simulink model "lqr_control_kalman_observer"  (R2020b)
settings: Solver=VariableStepAuto  StartTime=0.0  StopTime=30  RelTol=1e-3
undefined symbols (not defined in the file): A, B, C, C_discrete, D, D_discrete, DiscIntNeverNeededParam, Discrete, G, Gamma, h, h_plant, N, n, Phi, Q, Q0, Q1, Q2, R, R_discrete, reference, sat_max, sat_min, Time, wind_final_value, wind_initial_value, wind_steptime, x0
libraries: ctrlSharedLib x1
settings Model: Creator=lucas  LastModifiedBy=lucas

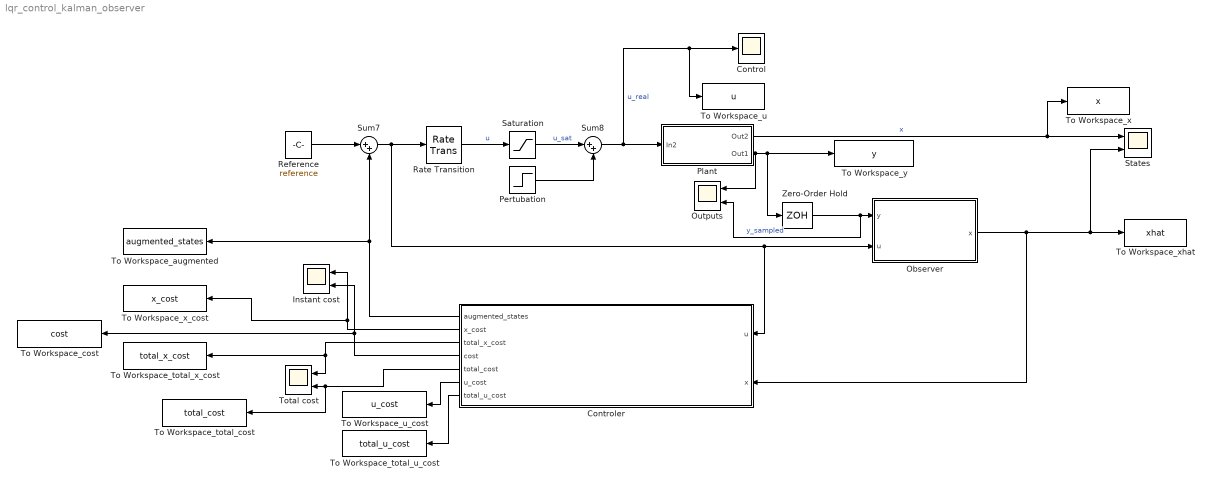
== system lqr_control_kalman_observer ==
  Control : Scope
  Controler : Subsystem
  Instant cost : Scope  NumInputPorts=2
  Observer : Subsystem
  Outputs : Scope  NumInputPorts=2
  Pertubation : Step  Time=wind_steptime  Before=wind_initial_value  After=wind_final_value  SampleTime=h_plant
  Plant : Subsystem
  Rate Transition : RateTransition  Integrity=off  OutPortSampleTimeMultiple=0.01  OutPortSampleTime=h_plant
  Reference : Constant  Value=reference  SampleTime=h
  Saturation : Saturate  UpperLimit=sat_max  LowerLimit=sat_min
  States : Scope  NumInputPorts=2
  Sum7 : Sum  Inputs=|++
  Sum8 : Sum  Inputs=|++
  To Workspace_augmented : ToWorkspace  VariableName=augmented_states  SaveFormat=Timeseries  SampleTime=-1
  To Workspace_cost : ToWorkspace  VariableName=cost  SaveFormat=Timeseries  SampleTime=-1
  To Workspace_total_cost : ToWorkspace  VariableName=total_cost  SaveFormat=Timeseries  SampleTime=-1
  To Workspace_total_u_cost : ToWorkspace  VariableName=total_u_cost  SaveFormat=Timeseries  SampleTime=-1
  To Workspace_total_x_cost : ToWorkspace  VariableName=total_x_cost  SaveFormat=Timeseries  SampleTime=-1
  To Workspace_u : ToWorkspace  VariableName=u  SaveFormat=Timeseries  SampleTime=-1
  To Workspace_u_cost : ToWorkspace  VariableName=u_cost  SaveFormat=Timeseries  SampleTime=-1
  To Workspace_x : ToWorkspace  VariableName=x  SaveFormat=Timeseries  SampleTime=-1
  To Workspace_x_cost : ToWorkspace  VariableName=x_cost  SaveFormat=Timeseries  SampleTime=-1
  To Workspace_xhat : ToWorkspace  VariableName=xhat  SaveFormat=Timeseries  SampleTime=-1
  To Workspace_y : ToWorkspace  VariableName=y  SaveFormat=Timeseries  SampleTime=-1
  Total cost : Scope  NumInputPorts=2
  Zero-Order Hold : ZeroOrderHold  SampleTime=h
  wires:
  Sum8/1 -> Plant/1(In2), To Workspace_u/1, Control/1  "u_real"
  Controler/4(cost) -> To Workspace_cost/1, Instant cost/2
  Sum7/1 -> Observer/2(u), Controler/1(u), Rate Transition/1
  Saturation/1 -> Sum8/1  "u_sat"
  Pertubation/1 -> Sum8/2
  Observer/1(x) -> Controler/2(x), To Workspace_xhat/1, States/2
  Plant/1(Out2) -> To Workspace_x/1, States/1  "x"
  Controler/5(total_cost) -> To Workspace_total_cost/1, Total cost/2
  Rate Transition/1 -> Saturation/1  "u"
  Controler/1(augmented_states) -> To Workspace_augmented/1, Sum7/2
  Reference/1 -> Sum7/1
  Zero-Order Hold/1 -> Observer/1(y), Outputs/2  "y_sampled"
  Plant/2(Out1) -> Outputs/1, To Workspace_y/1, Zero-Order Hold/1
  Controler/2(x_cost) -> To Workspace_x_cost/1, Instant cost/1
  Controler/6(u_cost) -> To Workspace_u_cost/1
  Controler/7(total_u_cost) -> To Workspace_total_u_cost/1
  Controler/3(total_x_cost) -> Total cost/1, To Workspace_total_x_cost/1

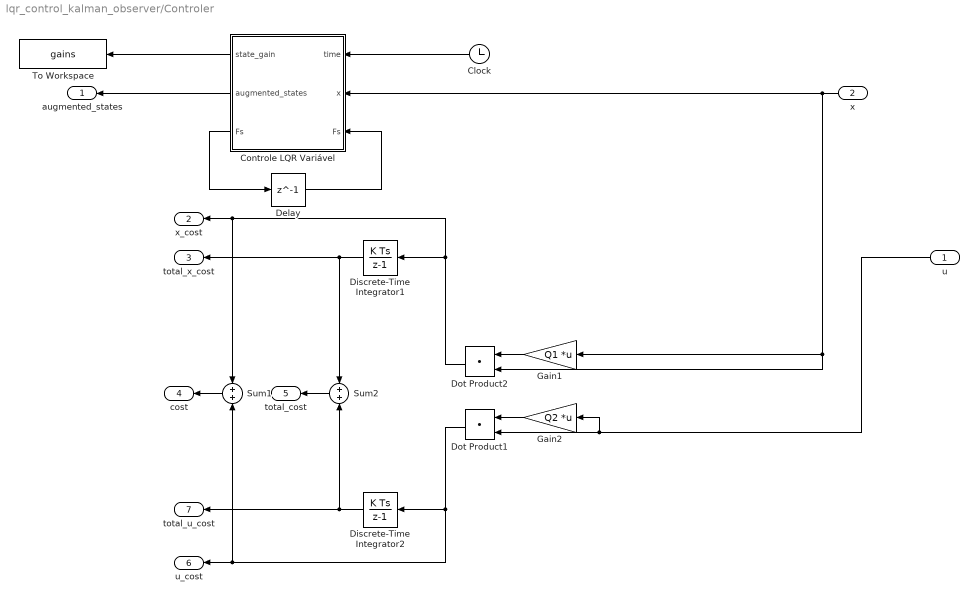
== system lqr_control_kalman_observer/Controler ==
  u : Inport
  x : Inport  Port=2
  Clock : Clock
  Controle LQR Variável : MATLAB Function  TreatAsAtomicUnit=on
  Delay : Delay  DelayLength=1  InitialCondition=zeros(1,n,1,N)  SampleTime=h
  Discrete-Time Integrator1 : DiscreteIntegrator  SampleTime=-1  ICPrevOutput=DiscIntNeverNeededParam  ICPrevScaledInput=DiscIntNeverNeededParam
  Discrete-Time Integrator2 : DiscreteIntegrator  SampleTime=-1  ICPrevOutput=DiscIntNeverNeededParam  ICPrevScaledInput=DiscIntNeverNeededParam
  Dot Product1 : DotProduct  InputSameDT=on  OutDataTypeStr=Inherit: Inherit via internal rule
  Dot Product2 : DotProduct  InputSameDT=on  OutDataTypeStr=Inherit: Inherit via internal rule
  Gain1 : Gain  Gain=Q1  Multiplication=Matrix(K*u)
  Gain2 : Gain  Gain=Q2  Multiplication=Matrix(K*u)
  Sum1 : Sum  Inputs=+|+
  Sum2 : Sum  Inputs=+|+
  To Workspace : ToWorkspace  VariableName=gains  SaveFormat=Timeseries  SampleTime=-1
  augmented_states : Outport
  x_cost : Outport  Port=2
  total_x_cost : Outport  Port=3
  cost : Outport  Port=4
  total_cost : Outport  Port=5
  u_cost : Outport  Port=6
  total_u_cost : Outport  Port=7
  wires:
  Gain1/1 -> Dot Product2/1
  u/1 -> Dot Product1/2, Gain2/1
  Dot Product2/1 -> Sum1/1, x_cost/1, Discrete-Time Integrator1/1
  Controle LQR Variável/2(augmented_states) -> augmented_states/1
  Gain2/1 -> Dot Product1/1
  Dot Product1/1 -> Discrete-Time Integrator2/1, Sum1/2, u_cost/1
  Discrete-Time Integrator1/1 -> total_x_cost/1, Sum2/1
  Discrete-Time Integrator2/1 -> Sum2/2, total_u_cost/1
  Sum1/1 -> cost/1
  Sum2/1 -> total_cost/1
  Controle LQR Variável/3(Fs) -> Delay/1
  Delay/1 -> Controle LQR Variável/3("Fs ")
  x/1 -> Dot Product2/2, Gain1/1, Controle LQR Variável/2(x)
  Controle LQR Variável/1(state_gain) -> To Workspace/1
  Clock/1 -> Controle LQR Variável/1(time)

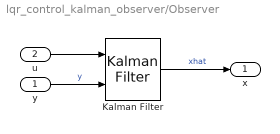
== system lqr_control_kalman_observer/Observer ==
  y : Inport
  u : Inport  Port=2
  Kalman Filter : ctrlSharedLib/Kalman Filter  TimeDomain=Discrete-Time  UseCurrentEstimator=on  ModelSource=Individual A, B, C, D matrices  ModelSourceVariable=ss(0.95,1,1,0,1)  A=Phi  B=Gamma  C=C_discrete  D=D_discrete  NumberOfStates=1  NumberOfInputs=1  NumberOfOutputs=1  InitialEstimateSource=Dialog  X0=0  P0=10  UseK=off  UseGH=on  NumberOfProcessNoiseInputs=1  G=G_discrete  TimeInvariantG=on  H=0  TimeInvariantH=on  Q=Q_discrete  TimeInvariantQ=on  R=R_discrete  TimeInvariantR=on  N=0  TimeInvariantN=on  AddInputPort=on  AddEnablePort=off  OutputEstimatedY=off  OutputP=off  Ts=h
  x : Outport
  wires:
  y/1 -> Kalman Filter/2  "y"
  u/1 -> Kalman Filter/1
  Kalman Filter/1 -> x/1  "xhat"

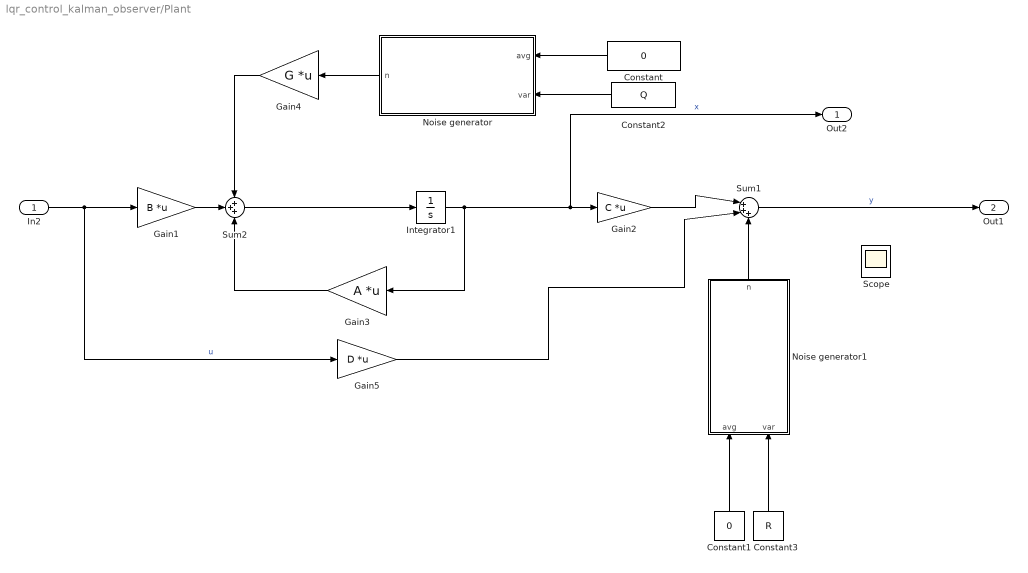
== system lqr_control_kalman_observer/Plant ==
  In2 : Inport
  Constant : Constant  Value=0  VectorParams1D=off
  Constant1 : Constant  Value=0
  Constant2 : Constant  Value=Q
  Constant3 : Constant  Value=R
  Gain1 : Gain  Gain=B  Multiplication=Matrix(K*u) (u vector)
  Gain2 : Gain  Gain=C  Multiplication=Matrix(K*u) (u vector)
  Gain3 : Gain  Gain=A  Multiplication=Matrix(K*u) (u vector)
  Gain4 : Gain  Gain=G  Multiplication=Matrix(K*u) (u vector)
  Gain5 : Gain  Gain=D  Multiplication=Matrix(K*u) (u vector)
  Integrator1 : Integrator  InitialCondition=x0
  Noise generator : MATLAB Function  TreatAsAtomicUnit=on
  Noise generator1 : MATLAB Function  TreatAsAtomicUnit=on
  Scope : Scope
  Sum1 : Sum  Inputs=|+++
  Sum2 : Sum  Inputs=+++
  Out2 : Outport
  Out1 : Outport  Port=2
  wires:
  Sum2/1 -> Integrator1/1
  Gain2/1 -> Sum1/1
  Sum1/1 -> Out1/1  "y"
  In2/1 -> Gain5/1, Gain1/1  "u"
  Integrator1/1 -> Gain3/1, Out2/1, Gain2/1  "x"
  Gain1/1 -> Sum2/2
  Gain3/1 -> Sum2/3
  Noise generator/1(n) -> Gain4/1
  Gain4/1 -> Sum2/1
  Constant/1 -> Noise generator/1(avg)
  Constant1/1 -> Noise generator1/1(avg)
  Constant3/1 -> Noise generator1/2(var)
  Constant2/1 -> Noise generator/2(var)
  Noise generator1/1(n) -> Sum1/3
  Gain5/1 -> Sum1/2

== matlab function lqr_control_kalman_observer/Controler/Controle LQR Variável ==
  settings: updateMethod=DISCRETE  sampleTime=h
  data: state_gain output; augmented_states output; Fs output; time input; x input; h parameter; n parameter; N parameter; Q0 parameter; Q1 parameter; Phi parameter; Gamma parameter; Q2 parameter; Fs input
function [state_gain, augmented_states, Fs]  = LQR(time, x, h, n, N, Q0, Q1, Phi, Gamma, Q2, Fs)
    idx = 1 + mod(floor(time/h),N);
    if (idx == 1)
        S = zeros(n,n,1,N+1);
        S(:,:,1,N+1) = Q0;
        for j=(N):-1:1
            first_val = Q1;
            second_val = (Phi' * S(:,:,1,j+1) * Phi);
            third_val = (Phi' * S(:,:,1,j+1) * Gamma)*(((Gamma' * S(:,:,1,j+1) * Gamma) + Q2)\(Gamma' * S(:,:,1,j+1) * Phi));
            S(:,:,1,j) = first_val + second_val - third_val;
            Fs(:,:,1,j) = ((Gamma' * S(:,:,1,j+1) * Gamma) + Q2)\(Gamma' * S(:,:,1,j+1) * Phi);
        end
    end
    state_gain = Fs(:,:,1,idx);
    augmented_states = -state_gain*x;

== matlab function lqr_control_kalman_observer/Plant/Noise generator1 ==
  data: avg input; n output; var input
function n = generate_gaussian_noise(avg, var)
n = avg + var*randn(length(var), 1);

== matlab function lqr_control_kalman_observer/Plant/Noise generator ==
  data: avg input; n output; var input
function n = generate_gaussian_noise(avg, var)
n = avg + var*randn(length(var), 1);
